simulink model "Task2simu"  (R2020b)
settings: Solver=VariableStepAuto  StartTime=0.0  StopTime=100.0  RelTol=1e-3
settings Model: Creator=CLINT  LastModifiedBy=CLINT

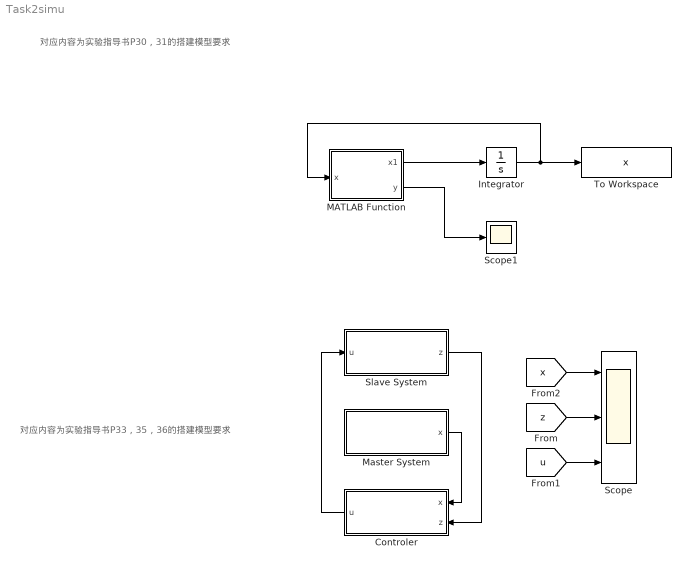
== system Task2simu ==
  note: 对应内容为实验指导书P30，31的搭建模型要求
  note: 对应内容为实验指导书P33，35，36的搭建模型要求
  Controler : Subsystem
  Integrator : Integrator  InitialCondition=[0.1;0.2;0.1]
  MATLAB Function : MATLAB Function  TreatAsAtomicUnit=on
  Master System : Subsystem
  Scope : Scope  NumInputPorts=3
  Scope1 : Scope
  Slave System : Subsystem
  To Workspace : ToWorkspace  VariableName=x  SaveFormat=Timeseries  SampleTime=-1
  wires:
  MATLAB Function/2(y) -> Scope1/1
  Integrator/1 -> To Workspace/1, MATLAB Function/1(x)
  MATLAB Function/1(x1) -> Integrator/1
  Controler/1(u) -> Slave System/1(u)
  [z] -> Scope/2
  Master System/1(x) -> Controler/1(x)
  Slave System/1(z) -> Controler/2(z)
  [x] -> Scope/1
  [u] -> Scope/3

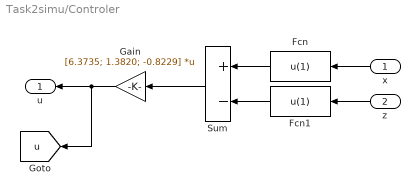
== system Task2simu/Controler ==
  x : Inport
  z : Inport  Port=2
  Fcn : Fcn  Expr=u(1)
  Fcn1 : Fcn  Expr=u(1)
  Gain : Gain  Gain=[6.3735; 1.3820; -0.8229]  Multiplication=Matrix(K*u)
  Sum : Sum  Inputs=+-
  u : Outport  VectorParamsAs1DForOutWhenUnconnected=off
  tag scope: u=global
  wires:
  x/1 -> Fcn/1
  z/1 -> Fcn1/1
  Sum/1 -> Gain/1
  Gain/1 -> [u], u/1
  Fcn/1 -> Sum/1
  Fcn1/1 -> Sum/2

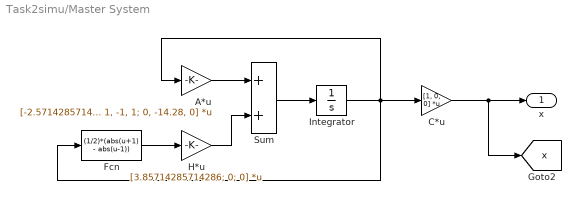
== system Task2simu/Master System ==
  A*u : Gain  Gain=[-2.57142857142857, 9, 0; 1, -1, 1; 0, -14.28, 0]  Multiplication=Matrix(K*u)
  C*u : Gain  Gain=[1, 0, 0]  Multiplication=Matrix(K*u)
  Fcn : Fcn  Expr=(1/2)*(abs(u+1) - abs(u-1))
  H*u : Gain  Gain=[3.85714285714286; 0; 0]  Multiplication=Matrix(K*u)
  Integrator : Integrator  InitialCondition=[-0.2; 0.3; 0.7]
  Sum : Sum
  x : Outport  VectorParamsAs1DForOutWhenUnconnected=off
  tag scope: x=global
  wires:
  A*u/1 -> Sum/1
  H*u/1 -> Sum/2
  Sum/1 -> Integrator/1
  Fcn/1 -> H*u/1
  C*u/1 -> [x], x/1
  Integrator/1 -> Fcn/1, C*u/1, A*u/1

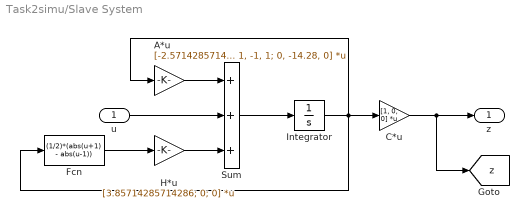
== system Task2simu/Slave System ==
  u : Inport
  A*u : Gain  Gain=[-2.57142857142857, 9, 0; 1, -1, 1; 0, -14.28, 0]  Multiplication=Matrix(K*u)
  C*u : Gain  Gain=[1, 0, 0]  Multiplication=Matrix(K*u)
  Fcn : Fcn  Expr=(1/2)*(abs(u+1) - abs(u-1))
  H*u : Gain  Gain=[3.85714285714286; 0; 0]  Multiplication=Matrix(K*u)
  Integrator : Integrator  InitialCondition=[-0.2; 0.3; 1]
  Sum : Sum  Inputs=+++
  z : Outport  VectorParamsAs1DForOutWhenUnconnected=off
  tag scope: z=global
  wires:
  H*u/1 -> Sum/3
  Fcn/1 -> H*u/1
  A*u/1 -> Sum/1
  u/1 -> Sum/2
  Sum/1 -> Integrator/1
  C*u/1 -> [z], z/1
  Integrator/1 -> Fcn/1, A*u/1, C*u/1

== matlab function Task2simu/MATLAB Function ==
  data: x input; x1 output; y output
function [x1,y] = fcn(x)
    x1 = zeros(3,1);
    a = 9;
    b = 14.28;
    c = 1;
    m0 = -1/7;
    m1 = 2/7;
    h = m1*x(1)+1/2*(m0-m1)*(abs(x(1)+c)-abs(x(1)-c));
    x1(1) = a*(x(2)-h);
    x1(2) = x(1)-x(2)+x(3);
    x1(3) = -b*x(2);
    y = x(1);
